simulink model "Harness"  (R2024b)
settings: Solver=VariableStepAuto  StartTime=0.0  StopTime=10.0  RelTol=1e-3
InitFcn:
  | init_fn;
libraries: simulink x8
settings Model: Creator=nan  LastModifiedBy=nan

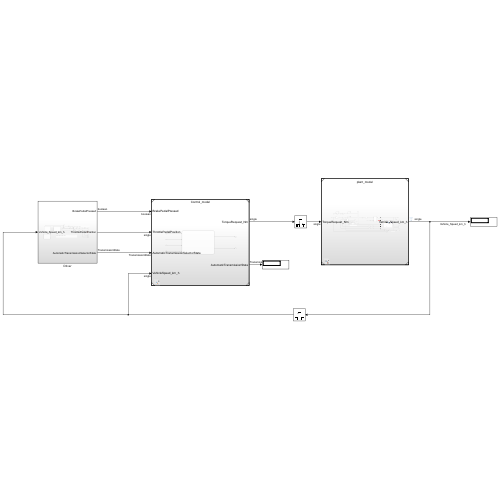
[thumbnail: Simulink's stored preview of the top-level diagram]
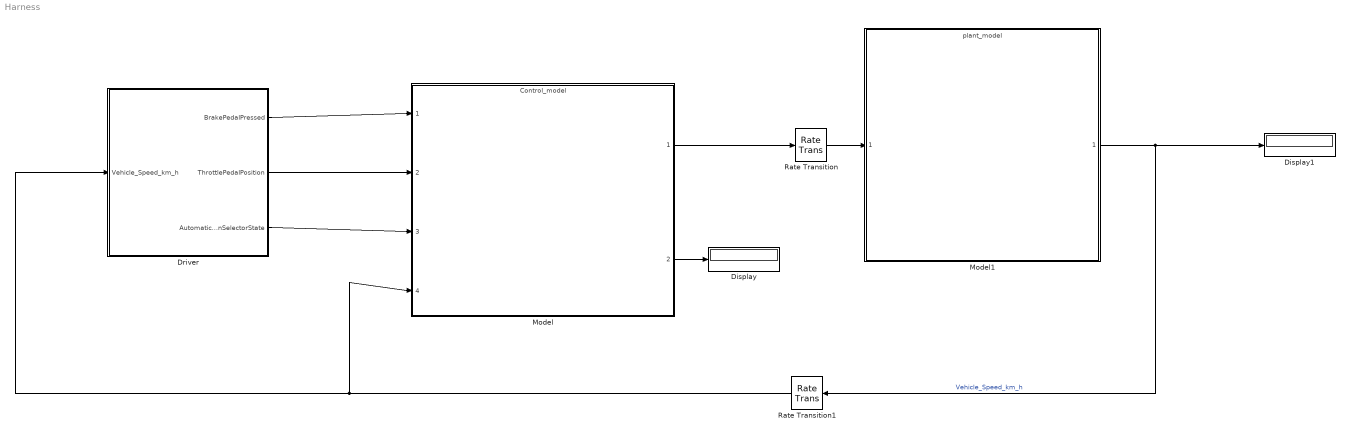
== system Harness ==
  Display : Display
  Display1 : Display
  Driver : Subsystem
  Model : ModelReference  ModelNameDialog=Control_model.slx  SimulationMode=Normal  ModelReferenceVersion=1.4
  Model1 : ModelReference  ModelNameDialog=plant_model.slx  SimulationMode=Normal  ModelReferenceVersion=1.4
  Rate Transition : RateTransition
  Rate Transition1 : RateTransition
  wires:
  Model/1 -> Rate Transition/1
  Rate Transition/1 -> Model1/1
  Model/2 -> Display/1
  Rate Transition1/1 -> Driver/1(Vehicle_Speed_km_h), Model/4
  Model1/1 -> Display1/1, Rate Transition1/1  "Vehicle_Speed_km_h"
  Driver/1(BrakePedalPressed) -> Model/1
  Driver/2(ThrottlePedalPosition) -> Model/2
  Driver/3(AutomaticTransmissionSelectorState) -> Model/3

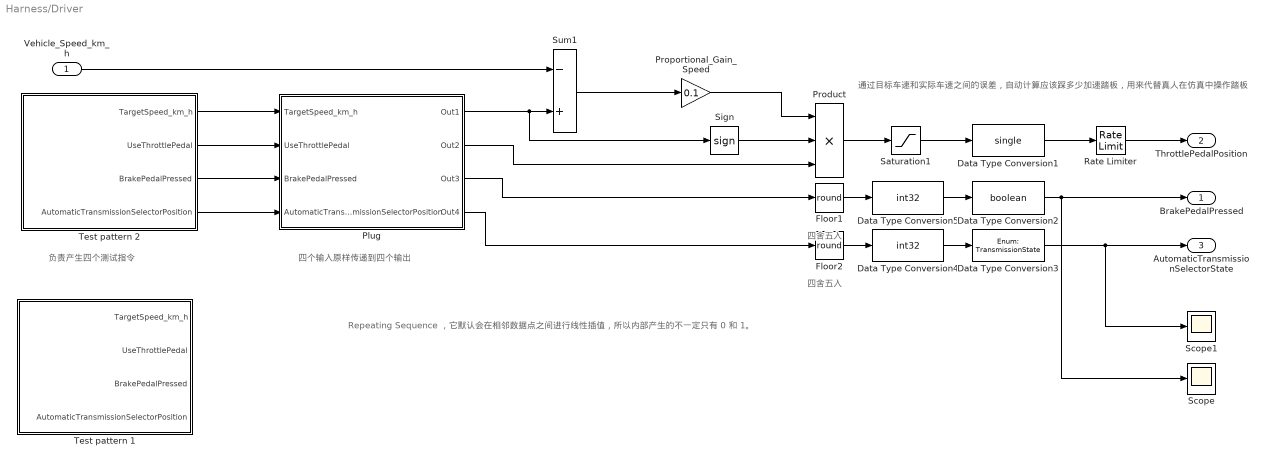
== system Harness/Driver ==
  note: 通过目标车速和实际车速之间的误差，自动计算应该踩多少加速踏板，用来代替真人在仿真中操作踏板
  note: Repeating Sequence ，它默认会在相邻数据点之间进行线性插值，所以内部产生的不一定只有 0 和 1。
  note: 四舍五入
  note: 四个输入原样传递到四个输出
  note: 负责产生四个测试指令
  note: 四舍五入
  Vehicle_Speed_km_h : Inport
  Data Type Conversion1 : DataTypeConversion  OutDataTypeStr=single  SaturateOnIntegerOverflow=off  RndMeth=Floor  LockScale=on
  Data Type Conversion2 : DataTypeConversion  OutDataTypeStr=boolean  SaturateOnIntegerOverflow=off  RndMeth=Floor  LockScale=on
  Data Type Conversion3 : DataTypeConversion  OutDataTypeStr=Enum: TransmissionState  SaturateOnIntegerOverflow=off  RndMeth=Floor  LockScale=on
  Data Type Conversion4 : DataTypeConversion  OutDataTypeStr=int32  SaturateOnIntegerOverflow=off  RndMeth=Floor  LockScale=on
  Data Type Conversion5 : DataTypeConversion  OutDataTypeStr=int32  SaturateOnIntegerOverflow=off  RndMeth=Floor  LockScale=on
  Floor1 : Rounding  Operator=round
  Floor2 : Rounding  Operator=round
  Plug : Subsystem
  Product : Product  Inputs=3
  Proportional_Gain_Speed : Gain  Gain=0.1
  Rate Limiter : RateLimiter  RisingSlewLimit=0.5  SampleTimeMode=inherited
  Saturation1 : Saturate  UpperLimit=1  LowerLimit=0
  Scope : Scope
  Scope1 : Scope
  Sign : Signum
  Sum1 : Sum  Inputs=-+
  Test pattern 1 : Subsystem
  Test pattern 2 : Subsystem
  BrakePedalPressed : Outport
  ThrottlePedalPosition : Outport  Port=2
  AutomaticTransmissionSelectorState : Outport  Port=3  OutDataTypeStr=Enum: TransmissionState
  wires:
  Test pattern 2/1(TargetSpeed_km_h) -> Plug/1(TargetSpeed_km_h)
  Test pattern 2/2(UseThrottlePedal) -> Plug/2(UseThrottlePedal)
  Test pattern 2/3(BrakePedalPressed) -> Plug/3(BrakePedalPressed)
  Test pattern 2/4(AutomaticTransmissionSelectorPosition) -> Plug/4(AutomaticTransmissionSelectorPosition)
  Vehicle_Speed_km_h/1 -> Sum1/1
  Saturation1/1 -> Data Type Conversion1/1
  Plug/1(Out1) -> Sign/1, Sum1/2
  Sum1/1 -> Proportional_Gain_Speed/1
  Product/1 -> Saturation1/1
  Data Type Conversion1/1 -> Rate Limiter/1
  Rate Limiter/1 -> ThrottlePedalPosition/1
  Proportional_Gain_Speed/1 -> Product/1
  Sign/1 -> Product/2
  Plug/2(Out2) -> Product/3
  Plug/3(Out3) -> Floor1/1
  Data Type Conversion5/1 -> Data Type Conversion2/1
  Data Type Conversion2/1 -> Scope/1, BrakePedalPressed/1
  Floor1/1 -> Data Type Conversion5/1
  Floor2/1 -> Data Type Conversion4/1
  Data Type Conversion3/1 -> Scope1/1, AutomaticTransmissionSelectorState/1
  Data Type Conversion4/1 -> Data Type Conversion3/1
  Plug/4(Out4) -> Floor2/1

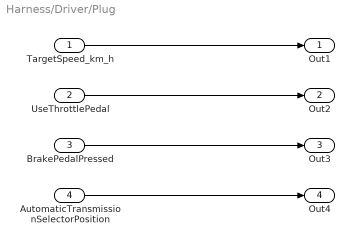
== system Harness/Driver/Plug ==
  TargetSpeed_km_h : Inport
  UseThrottlePedal : Inport  Port=2
  BrakePedalPressed : Inport  Port=3
  AutomaticTransmissionSelectorPosition : Inport  Port=4
  Out1 : Outport
  Out2 : Outport  Port=2
  Out3 : Outport  Port=3
  Out4 : Outport  Port=4
  wires:
  TargetSpeed_km_h/1 -> Out1/1
  UseThrottlePedal/1 -> Out2/1
  BrakePedalPressed/1 -> Out3/1
  AutomaticTransmissionSelectorPosition/1 -> Out4/1

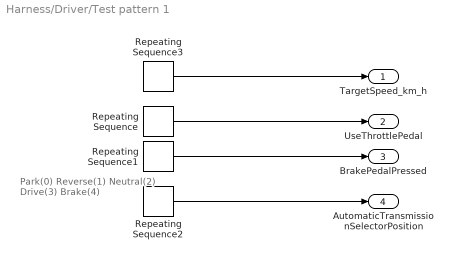
== system Harness/Driver/Test pattern 1 ==
  note: Park(0)
      | Reverse(1)
      | Neutral(2)
      | Drive(3)
      | Brake(4)
  Repeating Sequence : simulink/Sources/Repeating Sequence  rep_seq_t=[0 3.9 4 500]  rep_seq_y=[0 0 1 1]
  Repeating Sequence1 : simulink/Sources/Repeating Sequence  rep_seq_t=[0 2.999 3 49.9 50.0 52.0 52.1 500]  rep_seq_y=[1 1 0 0 1 1 0 0]
  Repeating Sequence2 : simulink/Sources/Repeating Sequence  rep_seq_t=[0 1.999 2 10 49.9 50.0 500]  rep_seq_y=[0 0 4 4 4 1 1]
  Repeating Sequence3 : simulink/Sources/Repeating Sequence  rep_seq_t=[0 3.9 4 29.9 30 39.9 40 52.9 53 500]  rep_seq_y=[0 0 90 90 60 60 0 0 -20 -20]
  TargetSpeed_km_h : Outport
  UseThrottlePedal : Outport  Port=2
  BrakePedalPressed : Outport  Port=3
  AutomaticTransmissionSelectorPosition : Outport  Port=4
  wires:
  Repeating Sequence2/1 -> AutomaticTransmissionSelectorPosition/1
  Repeating Sequence/1 -> UseThrottlePedal/1
  Repeating Sequence1/1 -> BrakePedalPressed/1
  Repeating Sequence3/1 -> TargetSpeed_km_h/1

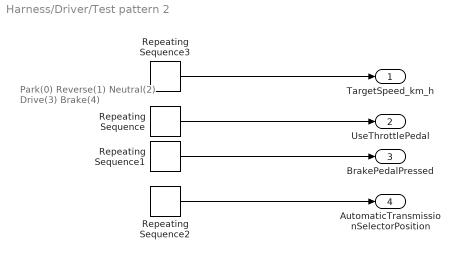
== system Harness/Driver/Test pattern 2 ==
  note: Park(0)
      | Reverse(1)
      | Neutral(2)
      | Drive(3)
      | Brake(4)
  Repeating Sequence : simulink/Sources/Repeating Sequence  rep_seq_t=[0 3.9 4 500]  rep_seq_y=[0 0 1 1]
  Repeating Sequence1 : simulink/Sources/Repeating Sequence  rep_seq_t=[0 2.999 3 49.9 80.0 82.0 92.1 500]  rep_seq_y=[1 1 0 0 1 1 0 0]
  Repeating Sequence2 : simulink/Sources/Repeating Sequence  rep_seq_t=[0 1.999 2 10 79.9 80.0 500]  rep_seq_y=[0 0 4 4 4 1 1]
  Repeating Sequence3 : simulink/Sources/Repeating Sequence  rep_seq_t=[0 3.9 4 29.9 30 39.9 40 82.9 83 500]  rep_seq_y=[0 0 90 90 60 60 0 0 -20 -20]
  TargetSpeed_km_h : Outport
  UseThrottlePedal : Outport  Port=2
  BrakePedalPressed : Outport  Port=3
  AutomaticTransmissionSelectorPosition : Outport  Port=4
  wires:
  Repeating Sequence2/1 -> AutomaticTransmissionSelectorPosition/1
  Repeating Sequence/1 -> UseThrottlePedal/1
  Repeating Sequence1/1 -> BrakePedalPressed/1
  Repeating Sequence3/1 -> TargetSpeed_km_h/1
